simulink model "modeloizaje"  (R2017a)
settings: Solver=VariableStepAuto  StartTime=0.0  StopTime=10.0  RelTol=1e-3
values from neighbouring files (symbols this model uses):
  Bheqd = (bh  + (beqd/(Rd^2)))    (= 32)    [datoscarro.m]
  Mheq = (Mh + (Jeqd/(Rd^2)))    (= 48014.2222222)    [datoscarro.m]
  Rd = 0.75    [datoscarro.m]
  rtd = 30    [datoscarro.m]
settings Model: Creator=tomas  LastModifiedBy=tomas

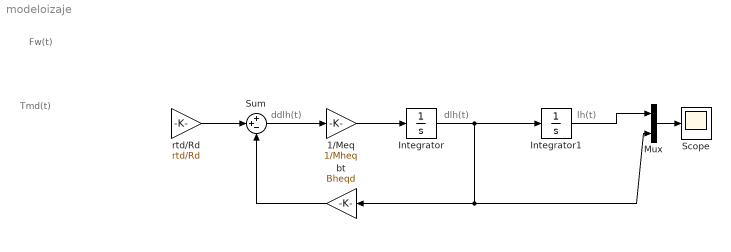
== system modeloizaje ==
  note: Fw(t)
  note: Tmd(t)
  note: ddlh(t)
  note: dlh(t)
  note: lh(t)
  1/Meq : Gain  Gain=1/Mheq
  Integrator : Integrator
  Integrator1 : Integrator
  Mux : Mux  Inputs=2
  Scope : Scope
  Sum : Sum  Inputs=++-
  bt : Gain  Gain=Bheqd
  rtd/Rd : Gain  Gain=rtd/Rd
  wires:
  Integrator1/1 -> Mux/1
  bt/1 -> Sum/3
  rtd/Rd/1 -> Sum/2
  Mux/1 -> Scope/1
  Sum/1 -> 1/Meq/1
  1/Meq/1 -> Integrator/1
  Integrator/1 -> Mux/2, bt/1, Integrator1/1
  ? -> rtd/Rd/1
  ? -> Sum/1
